simulink model "UAVSim"  (R2025b)
settings: Solver=FixedStepAuto  StartTime=0.0  StopTime=simTime  FixedStep=sampleTime  RelTol=1e-3
values from neighbouring files (symbols this model uses):
  blastParams = [thetaB_rad, phiB_rad, params.c, params.W, params.t0]    [main_optimize.m]
  CM = 0.1    [main_optimize.m]
  CT = m*g/4/rpm_nom^2    [main_optimize.m]
  desRPM = params.motorRPM*ones(4,1)    [main_optimize.m]
  dragConstsBody = -1/2*rho*bodyA*CD    [main_optimize.m]
  dragConstsMotor = -1/2*rho*motorA*CD    [main_optimize.m]
  g = 9.81    [main_optimize.m]
  m = mBody + 4*mMotor + 4*mArm    [main_optimize.m]
  quadDims = [rBody, rMotors, L]    [main_optimize.m]
  RMOTOR_iG = zeros(4,3)    [main_optimize.m]
  rpm2bodyMomentRollPitch = [-L L L -L ... (first row only)    [main_optimize.m]
  sampleTime = 0.0001    [main.m]    (also in main_compare.m)
libraries: aerolibobsolete x1, robotcorelib x1, aerolibutil x1, uavutilslib x1, dspsigops x1
settings Model: PauseTimes=1.23  SnapshotBufferSize=30  SnapshotInterval=1  Creator=root  LastModifiedBy=nkaka
settings DebuggingCC: ReadBeforeWriteMsg=DisableAll  WriteAfterWriteMsg=DisableAll  WriteAfterReadMsg=DisableAll  MultiTaskDSMMsg=none
settings ModelReferenceCC: UpdateModelReferenceTargets=IfOutOfDate
settings SFSimCC: SFSimEcho=off
settings RTWCC: GPUComputeCapability=3.5

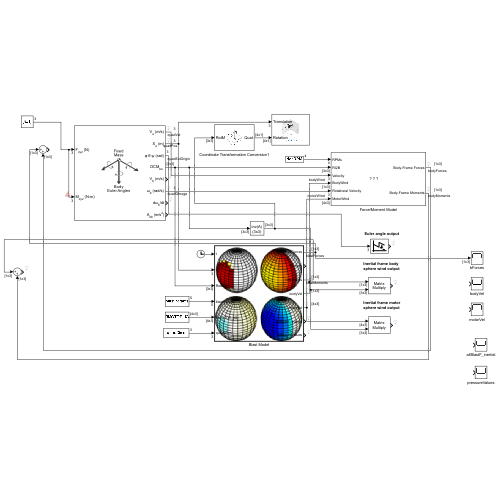
[thumbnail: Simulink's stored preview of the top-level diagram]
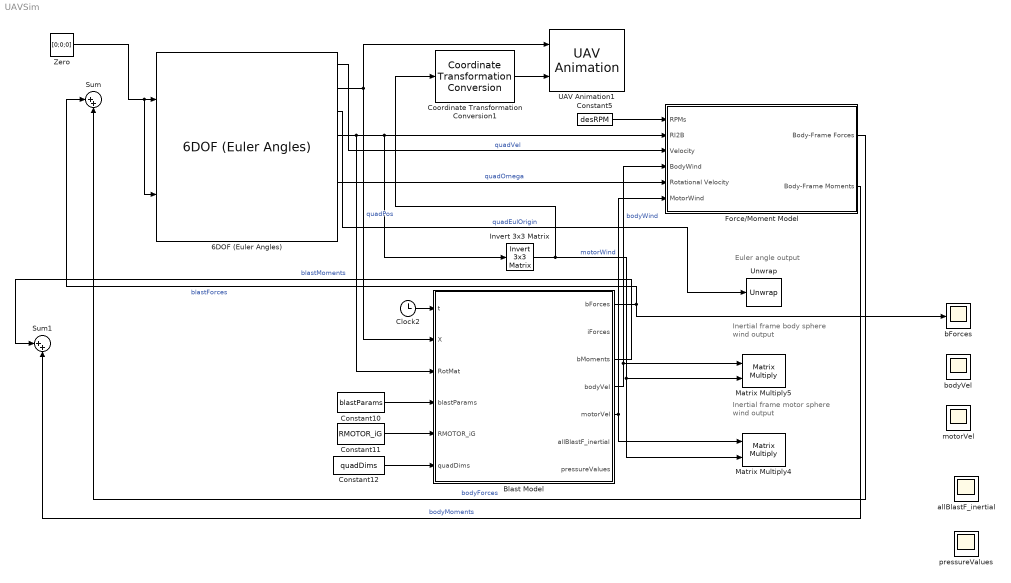
== system UAVSim ==
  note: Euler angle output
  note: Inertial frame body
      | sphere wind output
  note: Inertial frame motor
      | sphere wind output
  6DOF (Euler Angles) : aerolibobsolete/6DOF (Euler Angles)  units=Metric (MKS)  mtype=Fixed  rep=Euler Angles  xme_0=IC  Vm_0=[0 0 0]  eul_0=[0 0 0]  pm_0=[0 0 0]  mass_0=m  mass_e=0.5  mass_f=2.0  inertia=Iquad  inertia_e=eye(3)  inertia_f=2*eye(3)  k_quat=1.0  vre_flag=on  abi_flag=off  aMode=0  xme_statename=''  Vm_statename=''  eul_statename=''  quat_statename=''  pm_statename=''  mass_statename=''
  Blast Model : MATLAB Function  TreatAsAtomicUnit=on
  Clock2 : Clock
  Constant10 : Constant  Value=blastParams
  Constant11 : Constant  Value=RMOTOR_iG
  Constant12 : Constant  Value=quadDims
  Constant5 : Constant  Value=desRPM
  Coordinate Transformation Conversion1 : robotcorelib/Coordinate Transformation Conversion  InputRepresentation=Rotation Matrix  InputEulerSequence=ZYX  ShowTrVecInputPort=on  OutputRepresentation=Quaternion  OutputEulerSequence=ZYX  ShowTrVecOutputPort=on  SimulateUsing=Interpreted execution
      settings: LibrarySourceBlock=uavutilslib/Coordinate Transformation Conversion
  Force/Moment Model : Subsystem
      mask Display: image('simulinkImages/quad3dwithBlast.svg');
  Invert 3x3 Matrix : aerolibutil/Invert  3x3 Matrix
  Matrix Multiply4 : Product  Multiplication=Matrix(*)
  Matrix Multiply5 : Product  Multiplication=Matrix(*)
  Sum : Sum  Inputs=|++
  Sum1 : Sum  Inputs=|++
  UAV Animation1 : uavutilslib/UAV Animation  NumUAV=1  DynamicUAVConfig=off  UAVType=Multirotor  UAVSize=1  UAVColor=[1 0 0]  UAVTrajectoryAlpha=1  InertialZDirection=Down  RotationFormat=Quaternion  DrawMarkers=off  SampleTime=sampleTime
  Unwrap : dspsigops/Unwrap  tol=pi  running=off
  Zero : Constant  Value=[0;0;0]  OutDataTypeStr=Inherit: Inherit via back propagation
  allBlastF_inertial : Scope
      settings: DataLoggingVariableName=ScopeData3
  bForces : Scope
  bodyVel : Scope
  motorVel : Scope
      settings: DataLoggingVariableName=ScopeData2
  pressureValues : Scope
      settings: DataLoggingVariableName=ScopeData4
  wires:
  Blast Model/1(bForces) -> Sum/1, bForces/1  "blastForces"
  6DOF (Euler Angles)/1 -> Force/Moment Model/3(Velocity)  "quadVel"
  Clock2/1 -> Blast Model/1(t)
  6DOF (Euler Angles)/6 -> Force/Moment Model/5(Rotational Velocity)  "quadOmega"
  6DOF (Euler Angles)/2 -> Blast Model/2(X), UAV Animation1/1  "quadPos"
  6DOF (Euler Angles)/3 -> Unwrap/1  "quadEulOrigin"
  6DOF (Euler Angles)/4 -> Force/Moment Model/2(RI2B), Invert 3x3 Matrix/1, Blast Model/3(RotMat)
  Constant10/1 -> Blast Model/4(blastParams)
  Constant11/1 -> Blast Model/5(RMOTOR_iG)
  Constant12/1 -> Blast Model/6(quadDims)
  Constant5/1 -> Force/Moment Model/1(RPMs)
  Invert 3x3 Matrix/1 -> Matrix Multiply4/2, Matrix Multiply5/2, Coordinate Transformation Conversion1/1
  Blast Model/3(bMoments) -> Sum1/1  "blastMoments"
  Force/Moment Model/1(Body-Frame Forces) -> Sum/2  "bodyForces"
  Blast Model/4(bodyVel) -> Force/Moment Model/4(BodyWind), Matrix Multiply5/1  "bodyWind"
  Force/Moment Model/2(Body-Frame Moments) -> Sum1/2  "bodyMoments"
  Blast Model/5(motorVel) -> Matrix Multiply4/1, Force/Moment Model/6(MotorWind)  "motorWind"
  Coordinate Transformation Conversion1/1 -> UAV Animation1/2
  Zero/1 -> 6DOF (Euler Angles)/2, 6DOF (Euler Angles)/1

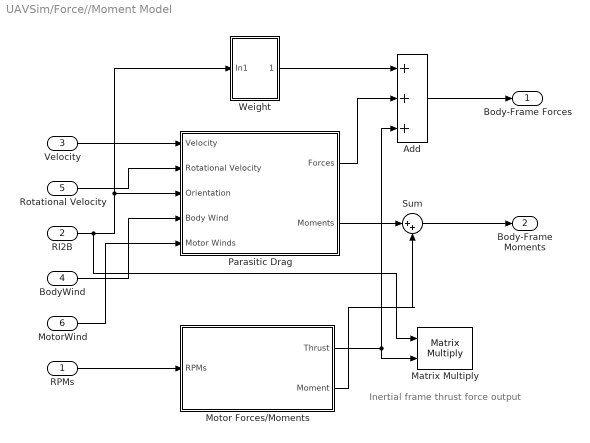
== system UAVSim/Force//Moment Model ==
  note: Inertial frame thrust force output
  RPMs : Inport
  RI2B : Inport  Port=2
  Velocity : Inport  Port=3
  BodyWind : Inport  Port=4
  Rotational Velocity : Inport  Port=5
  MotorWind : Inport  Port=6
  Add : Sum  Inputs=+++
  Matrix Multiply : Product  Multiplication=Matrix(*)
  Motor Forces/Moments : Subsystem
  Parasitic Drag : Subsystem
  Sum : Sum  Inputs=|++
  Weight : Subsystem
  Body-Frame Forces : Outport
  Body-Frame Moments : Outport  Port=2
  wires:
  RPMs/1 -> Motor Forces/Moments/1(RPMs)
  Rotational Velocity/1 -> Parasitic Drag/2(Rotational Velocity)
  Velocity/1 -> Parasitic Drag/1(Velocity)
  MotorWind/1 -> Parasitic Drag/5(Motor Winds)
  BodyWind/1 -> Parasitic Drag/4(Body Wind)
  RI2B/1 -> Weight/1(In1), Parasitic Drag/3(Orientation), Matrix Multiply/1
  Weight/1(Out1) -> Add/1
  Parasitic Drag/1(Forces) -> Add/2
  Parasitic Drag/2(Moments) -> Sum/1
  Motor Forces/Moments/1(Thrust) -> Matrix Multiply/2, Add/3
  Motor Forces/Moments/2(Moment) -> Sum/2
  Add/1 -> Body-Frame Forces/1
  Sum/1 -> Body-Frame Moments/1

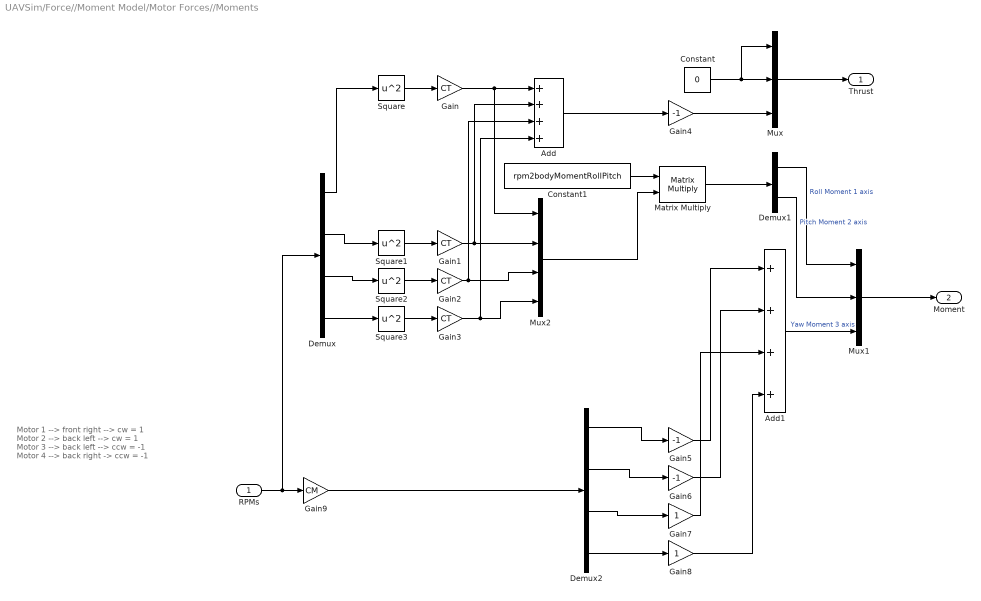
== system UAVSim/Force//Moment Model/Motor Forces//Moments ==
  note: Motor 1 --> front right --> cw = 1
      | Motor 2 --> back left --> cw = 1
      | Motor 3 --> back left --> ccw = -1
      | Motor 4 --> back right -> ccw = -1
  RPMs : Inport
  Add : Sum  Inputs=++++
  Add1 : Sum  Inputs=++++
  Constant : Constant  Value=0
  Constant1 : Constant  Value=rpm2bodyMomentRollPitch
  Demux : Demux
  Demux1 : Demux  Outputs=2
  Demux2 : Demux
  Gain{,1..3} (4 alike) : Gain  Gain=CT
  Gain4 : Gain  Gain=-1
  Gain5 : Gain  Gain=-1
  Gain6 : Gain  Gain=-1
  Gain7 : Gain
  Gain8 : Gain
  Gain9 : Gain  Gain=CM
  Matrix Multiply : Product  Multiplication=Matrix(*)
  Mux : Mux  Inputs=3
  Mux1 : Mux  Inputs=3
  Mux2 : Mux
  Square{,1..3} (4 alike) : Math  Operator=square
  Thrust : Outport
  Moment : Outport  Port=2
  wires:
  RPMs/1 -> Demux/1, Gain9/1
  Demux/1 -> Square/1
  Demux/2 -> Square1/1
  Demux2/1 -> Gain5/1
  Demux/3 -> Square2/1
  Square2/1 -> Gain2/1
  Gain9/1 -> Demux2/1
  Constant/1 -> Mux/2, Mux/1
  Demux/4 -> Square3/1
  Square/1 -> Gain/1
  Square1/1 -> Gain1/1
  Gain/1 -> Mux2/1, Add/1
  Square3/1 -> Gain3/1
  Gain1/1 -> Mux2/2, Add/2
  Gain2/1 -> Add/3, Mux2/3
  Gain3/1 -> Add/4, Mux2/4
  Add/1 -> Gain4/1
  Constant1/1 -> Matrix Multiply/1
  Mux2/1 -> Matrix Multiply/2
  Demux2/2 -> Gain6/1
  Demux2/3 -> Gain7/1
  Demux2/4 -> Gain8/1
  Gain4/1 -> Mux/3
  Matrix Multiply/1 -> Demux1/1
  Demux1/2 -> Mux1/2  "Pitch Moment 2 axis"
  Gain5/1 -> Add1/1
  Gain6/1 -> Add1/2
  Gain7/1 -> Add1/3
  Gain8/1 -> Add1/4
  Mux/1 -> Thrust/1
  Demux1/1 -> Mux1/1  "Roll Moment 1 axis"
  Add1/1 -> Mux1/3  "Yaw Moment 3 axis"
  Mux1/1 -> Moment/1

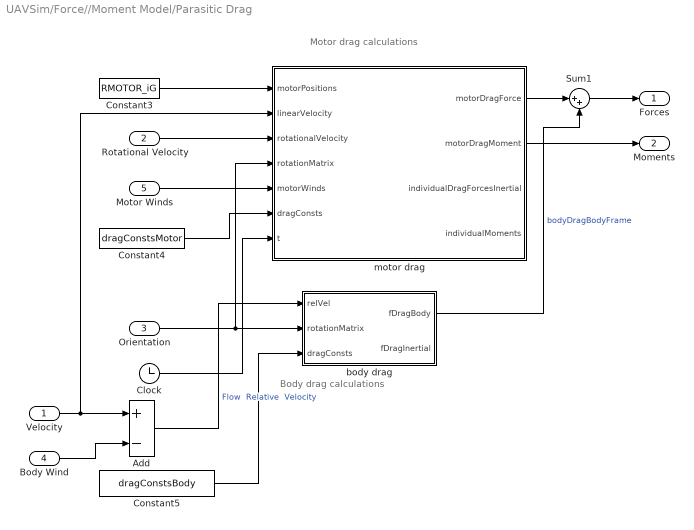
== system UAVSim/Force//Moment Model/Parasitic Drag ==
  note: Motor drag calculations
  note: Body drag calculations
  Velocity : Inport
  Rotational Velocity : Inport  Port=2
  Orientation : Inport  Port=3
  Body Wind : Inport  Port=4
  Motor Winds : Inport  Port=5
  Add : Sum  Inputs=+-
  Clock : Clock
  Constant3 : Constant  Value=RMOTOR_iG
  Constant4 : Constant  Value=dragConstsMotor
  Constant5 : Constant  Value=dragConstsBody
  Sum1 : Sum  Inputs=|++
  body drag : MATLAB Function  TreatAsAtomicUnit=on
  motor drag : MATLAB Function  TreatAsAtomicUnit=on
  Forces : Outport
  Moments : Outport  Port=2
  wires:
  Orientation/1 -> motor drag/4(rotationMatrix), body drag/2(rotationMatrix)
  Velocity/1 -> Add/1, motor drag/2(linearVelocity)
  Constant4/1 -> motor drag/6(dragConsts)
  Motor Winds/1 -> motor drag/5(motorWinds)
  body drag/1(fDragBody) -> Sum1/2  "bodyDragBodyFrame"
  Body Wind/1 -> Add/2
  Clock/1 -> motor drag/7(t)
  Constant5/1 -> body drag/3(dragConsts)
  Rotational Velocity/1 -> motor drag/3(rotationalVelocity)
  Constant3/1 -> motor drag/1(motorPositions)
  Add/1 -> body drag/1(relVel)  "Flow  Relative  Velocity"
  motor drag/1(motorDragForce) -> Sum1/1
  motor drag/2(motorDragMoment) -> Moments/1
  Sum1/1 -> Forces/1

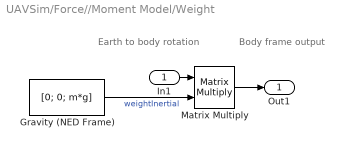
== system UAVSim/Force//Moment Model/Weight ==
  note: Earth to body rotation
  note: Body frame output
  In1 : Inport
  Gravity (NED Frame) : Constant  Value=[0; 0; m*g]
  Matrix Multiply : Product  Multiplication=Matrix(*)
  Out1 : Outport
  wires:
  Gravity (NED Frame)/1 -> Matrix Multiply/2  "weightInertial"
  In1/1 -> Matrix Multiply/1
  Matrix Multiply/1 -> Out1/1

== matlab function UAVSim/Blast Model ==
  data: t input; X input double; bForces output double [-500000..500000]; iForces output; RotMat input; blastParams input; RMOTOR_iG input; quadDims input; bMoments output double [-500000..500000]; bodyVel output double; motorVel output double; allBlastF_inertial output; pressureValues output
function [bForces, iForces, bMoments, bodyVel, motorVel, allBlastF_inertial, pressureValues] = blastFMCalc(t, X, RotMat, blastParams, RMOTOR_iG, quadDims)
%% Inputs:
% t = current sim time
% X = current quad position
% RotMat = current quad orientation matrix earth to body frame
% blastParams = [Time of hit, Overpressure, theta, psi, tau, c] = [t, Ps, theta, psi, tau, c]
% RMOTOR_iG = Motor positions = [rBody, rMotors, rMotors, rMotors, rMotors]
% quadDims = Quadrotor dimensions = [rBody, rMotors, L]
% onOff = toggle for enabling the blasts in the simulink simulation

%% Initialize outputs
bForces = zeros(1,3);
iForces = zeros(1,3);
bMoments = zeros(1,3);
bodyVel = zeros(1,3);
motorVel = zeros(4,3);
allBlastF_inertial = zeros(5,3);
pressureValues = zeros(5,100);
onOffPressure = 1;
onOffVelocity = 1;
mach2ms = 343;

%% Unpack quadrotor dimensions
rBody = quadDims(1);
rMotors = quadDims(2);

%% Make the rotation matrix more clear
Rb2i = RotMat';
Ri2b = RotMat;

%% Get blast parameters
t0 = blastParams(5);
theta = blastParams(1); % Elevation
phi = blastParams(2); % Azimuth
ccccccccc = blastParams(3);
W = blastParams(4);

% Best fit c function
% cF = 
% 
%      General model Power2:
%      cF(x) = a*x^b+c
%      Coefficients (with 95% confidence bounds):
%        a =        1698  (1687, 1709)
%        b =     -0.6454  (-0.6496, -0.6413)
%        c =       73.96  (67.94, 79.98)
function c = cF(x)
    c = 1698*abs(x)^(-0.6454) + 73.96;
end

% Calculate vector for orientation of the blast, opposite of NED to get the intended effect
vec = [sin(phi)*cos(theta), sin(phi)*sin(theta), cos(phi)]*Ri2b;

%% Setup Sadovskiy models for tau and Ps
function [sadPs, sadTau] = sadovskiy(WW,RR)
% Check that RR is positive
assert(RR >= 0);

% Set common consts
crW = WW^(1/3);
kgcmsq2pa = 98066.5;

% Calculate values from Sadovisky
sadTau = nthroot(WW,6)*sqrt(RR)/1000; % converted to seconds
sadPs = (0.95*(crW/RR) + 3.9*((crW/RR)^2) + 13*((crW/RR)^3))*kgcmsq2pa;
end

%% Setup heaviside function since the default matlab one won't work with code gen
function H = heavisideFcn(X)
    % https://en.wikipedia.org/wiki/Heaviside_step_function
    H = zeros(size(X));
    for iii = 1:length(X)
        if X(iii) >= 0
            H(iii) = 1;
        % else
        %     H(i) = 0;
        end
    end
end

%% Setup a rounding function for rounding to a particular decimal place with code-gen
function out = round2Digits(in,decs)
% https://www.mathworks.com/matlabcentral/answers/17598-how-to-convert-a-string-to-int
roundingNum = str2double(append('1',repmat(['0'],1,decs-1)));
out = round(in.*roundingNum)./roundingNum;
end

%% Setup the dewey parameter interpolation functions
function [v,alpha,beta,a,tstar] = deweyParams(scaledDist)
%% Function info:
% Inputs:
%      scaledDist = d/S = double
%          d = distance from blast
%          S = (W*P0/P)^(1/3)
%               W = weight of explosive used in blast
%               P0 = standard pressure = 101.325
%               P = ambient pressure
%
% Outputs:
%      v = peak velocity (m/s), converted from mach
%      alpha = unitless fitted parameter
%      beta = unitless fitted parameter
%      a = unitless fitted parameter
%      tstar = unitless fitted parameter

%% Setup the dewey parameter interpolation functions
% Set functions for interpolating the parameters, with their derivatives
function out = vMachFcn(xx,option)
    if option == 1
        vMach1 = 6.38*xx^-1.51;
        out = vMach1;
    elseif option == 2
        vMachDer = (-1.51*6.38)*xx^(-1.51-1);
        out = vMachDer;
    else
        error('Choose a valid output option')
    end
end

function out = alphaFcn(xx, option)
    if option == 1
        alpha1 = 1.5*xx^-0.926; % power series
        out = alpha1;
    elseif option == 2
        alphaDer = (-0.926*1.5)*xx^(-0.926-1);
        out = alphaDer;
    else
        error('Choose a valid output option')
    end
end

function out = betaFcn(xx,option)
    if option == 1
        beta1 = 1.64*xx^(-0.241); % Power
        out = beta1;
    elseif option == 2
        betaDer = (-0.241*1.64)*xx^(-0.241-1);
        out = betaDer;
    else
        error('Choose a valid output option')
    end
end

function out = aFcn(xx,option)
    if option == 1
        a1 = 1.95*xx^-1.02; % power series
        out = a1;
    elseif option == 2
        aDer = (-1.02*1.95)*xx^(-1.02-1);
        out = aDer;
    else
        error('Choose a valid output option')
    end
end

function out = tstarFcn(xx,option)
    if option == 1
        tstar1 = -0.326+0.93*log(max(1e-10, xx)); % Log
        out = tstar1;
    elseif option == 2
        tstarDer = 0.93/xx;
        out = tstarDer;
    else
        error('Choose a valid output option')
    end
end

% Set point to swtich from fitted curves to linear extrapolation for power series fits
xpt = 1.983489191;

% Set scaleDist to x for readability
xx = scaledDist;

% Peak velocity value - power series/ linear piecewise interpolation
if xx >= xpt
    % Regular interp function
    vMach = vMachFcn(xx,1);
else
    % Linear interp function
    yVal = vMachFcn(xpt,1);
    slope = vMachFcn(xpt,2);
    yIntercept = yVal - slope*xpt;
    vMach = slope*xx + yIntercept;
end
v = vMach;

% Alpha - power series/ linear piecewise interpolation
if xx >= xpt
    % Regular interp function
    alpha = alphaFcn(xx,1);
else
    % Linear interp function
    yVal = alphaFcn(xpt,1);
    slope = alphaFcn(xpt,2);
    yIntercept = yVal - slope*xpt;
    alpha = slope*xx + yIntercept;
end

% Beta - linear interpolation
if xx >= xpt
    % Regular interp function
    beta = betaFcn(xx,1);
else
    % Linear interp function
    yVal = betaFcn(xpt,1);
    slope = betaFcn(xpt,2);
    yIntercept = yVal - slope*xpt;
    beta = slope*xx + yIntercept;
end

% a - power series/ linear piecewise interpolation
if xx >= xpt
    % Regular interp function
    a = aFcn(xx,1);
else
    % Linear interp function
    yVal = aFcn(xpt,1);
    slope = aFcn(xpt,2);
    yIntercept = yVal - slope*xpt;
    a = slope*xx + yIntercept;
end

% tstar - linear interpolation
if xx >= xpt
    % Regular interp function
    tstar = tstarFcn(xx,1);
else
    % Linear interp function
    yVal = tstarFcn(xpt,1);
    slope = tstarFcn(xpt,2);
    yIntercept = yVal - slope*xpt;
    tstar = slope*xx + yIntercept;
end

end

%% Update outputs if onOff is true
if onOffPressure == 1
    %% Set sphere sizes and distances from center of blast
    d = -vecnorm(X);
    x = [linspace(-rBody,rBody);
         linspace(-rMotors,rMotors);
         linspace(-rMotors,rMotors);
         linspace(-rMotors,rMotors);
         linspace(-rMotors,rMotors)] + d;
    n = height(x);
    ds = zeros(n,1);
    for i = 1:n
        if i == 1
            ds(i) = vecnorm(X');
        else
            ds(i) = vecnorm(X'-RMOTOR_iG(i-1,:));
        end
    end

    %% Get the forces based on the desired times and overpressure values
    Fp = zeros(n,3);
    V = zeros(n,3);

    %% Get curret pressure at x1
    pp = zeros(size(x));
    for j = 1:n
        % Set radius
        if j == 1
            R = rBody;
            x0 = d - R;
        else
            R = rMotors;
            dTmp = vecnorm(X'-RMOTOR_iG(j-1,:));
            x0 = -dTmp - R;
        end
        [Ps, tau] = sadovskiy(W,ds(j));
    
        % Calculate pressure for this time step
        % val = t-(x(j,:)-x0)/ccccccccc;
        val = t-(x(j,:)-x0)/cF(d);
        Dt = val-t0;
        expr = Dt./tau;
        hval = heavisideFcn(Dt);
        pp(j,:) = Ps.*exp(-expr).*(1-expr).*hval;

        %% Calculate velocity based on modified Dewey model
        if onOffVelocity == 1
            % Get Dt
            ti = t;
            DT = ti-t0;
        
            % Calcualte scaled distance
            % val = t-(x(j,:)-x0)/ccccccccc;
            val = t-(x(j,:)-x0)/cF(d);
            Dt = val-t0; 
            hval = heavisideFcn(Dt);
            S = W^(1/3);
            scaledDist = ds(j)/S;
            % hval = heavisideFcn(ti-t0);
            % scaledTime = ccccccccc*DT/S;
            scaledTime = cF(d)*DT/S;

            % Get dewey params
            [Vs_i, alpha_i, beta_i, a_i, ~] = deweyParams(scaledDist);

            % Calculate velocity
            logVal = 1 + beta_i*scaledTime;
            if logVal < 0
                1;
            end
            % V(j,:) = (mach2ms * ((Vs_i*(1-beta_i*scaledTime) * exp(-alpha_i*scaledTime) + a_i*log(1 + beta_i*scaledTime)) * exp(-scaledTime)*ceil(sum(hval)/length(hval))))*vec;
            logVal = max(1e-10, 1 + beta_i*scaledTime);
            V(j,:) = (mach2ms * ((Vs_i*(1-beta_i*scaledTime) * exp(-alpha_i*scaledTime) + a_i*log(logVal)) * exp(-scaledTime)*ceil(sum(hval)/length(hval))))*vec;
           
        end
        if any(isnan(V))
            1;
        end
        roundedV = real(round2Digits(V,5)); % added real(.) here because otherwise simulink thinks that V could be complex due to it inheriting a variable that was once square rooted.............
        if any(isnan(roundedV))
            1;
        end
    end
    pressureValues = pp;
    
    %% Get current force due to pressure based on x1
    eps = 0.0000001;
    for j = 1:n
        % Set radius
        if j == 1
            R = rBody;
        else
            R = rMotors;
        end
    
        % Set current x and pp values
        currX = x(j,:);
        currPP = pp(j,:);

        % Calculate force
        sqrtVal = (R + eps)^2+(currX-d).^2;
        if any(sqrtVal < 0)
            1;
        end
        Fp(j,:) = ((trapz(currX-d,currPP.*(currX-d).*sqrt(sqrtVal))*-pi/R).*vec);
    end

    %% Output the velocities
    bodyVel = roundedV(1,:);
    motorVel = roundedV(2:5,:);

    %% Calculate total force due to the blast
    bForces = sum(Fp,1);
    iForces = bForces*Rb2i;
    
    %% Calculate resultant moment from blast
    Mblast = zeros(n-1,3);
    for j = 2:n
        Mblast(j-1,:) = cross(RMOTOR_iG(j-1,:),Fp(j,:));
    end
    bMoments = sum(Mblast,1);

    % Output full matrix of blast forces and moments
    allBlastF_inertial = Fp*Rb2i;
end

assert(~anynan(bForces) || allfinite(bForces))
assert(~anynan(iForces) || allfinite(iForces))
assert(~anynan(bMoments) || allfinite(bMoments))
assert(~anynan(bodyVel) || allfinite(bodyVel))
assert(~anynan(motorVel) || allfinite(motorVel))
assert(~anynan(allBlastF_inertial) || allfinite(allBlastF_inertial))


end

== matlab function UAVSim/Force//Moment Model/Parasitic Drag/motor drag ==
  data: motorPositions input; motorDragForce output; linearVelocity input; rotationalVelocity input; rotationMatrix input; motorDragMoment output; motorWinds input; dragConsts input; t input; individualDragForcesInertial output; individualMoments output
function [motorDragForce,motorDragMoment,individualDragForcesInertial,individualMoments] = motorDragCalc(motorPositions, linearVelocity, rotationalVelocity, rotationMatrix, motorWinds, dragConsts, t)
% Function to calculate the drag force and moments for the motors
% Inputs: 
%      motorPositions = Matrix of four position vectors denoting the position of each motor relative to the body (4,3)
%      linearVelocity = Linear velocity vector of the drone (1,3)
%      rotationalVelocity = Rotational velocity vector of the drone (1,3)
%      rotationMatrix = Orientation matrix of the drone (3,3) - inertial to body frame
%      motorWinds = wind experienced at each motor position (4,3)
%      dragConsts = -1/2 * rho * C_D * motorA
%
% Outputs:
%      motorDragForce = vector of total drag force on all motors (BODY FRAME)
%      motorDragMoment = vector of total drag moment caused by the wind-relative velocity on each motor (BODY FRAME)

%% Set output sizes
motorDragForce = zeros(1,3);
motorDragMoment = zeros(1,3);
individualDragForcesInertial = zeros(4,3);
individualMoments = zeros(4,3);

%% Set variables for readability
v = linearVelocity;
W = rotationalVelocity;
Rb2i = rotationMatrix';
Ri2b = rotationMatrix;
r_iG = motorPositions;

%% Calculate individual motor velocities
% Inertial velocity at each element
vmotor_iG = zeros(4,3);
vRelmotor_iG = zeros(4,3);
fDrag = zeros(4,3);
mDrag = zeros(4,3);
for i = 1:4
    vmotor_iG(i,:) = (v + (Rb2i*cross(r_iG(i,:),W)'));
    vRelmotor_iG(i,:) = vmotor_iG(i,:) - (Ri2b*motorWinds(i,:)')';
    vTmp = vRelmotor_iG(i,:);
    vecNorm = vecnorm(vTmp);

    % Calculate drag in the inertial frame, but output in the body frame
    fDrag(i,:) = (Ri2b*(dragConsts*vecNorm.*vTmp'))';

    % Calculate the drag momenet in the body frame
    mDrag(i,:) = cross(fDrag(i,:),r_iG(i,:));
end

%% Output force and moments
motorDragForce = sum(fDrag,1);
individualDragForcesInertial = fDrag*Rb2i;
motorDragMoment = sum(mDrag,1);
individualMoments = mDrag;

end

== matlab function UAVSim/Force//Moment Model/Parasitic Drag/body drag ==
  data: relVel input; fDragBody output; rotationMatrix input; dragConsts input; fDragInertial output
function [fDragBody, fDragInertial] = bodyDragCalc(relVel, rotationMatrix, dragConsts)
% Initialize
fDragBody = zeros(1,3);
fDragInertial = zeros(1,3);

% Unpack
Rb2i = rotationMatrix';
Ri2b = rotationMatrix;

% Calculate
vecNorm = sqrt(sum(conj(relVel).*relVel));
fDragBody = dragConsts*vecNorm.*relVel*Rb2i;
fDragInertial = fDragBody*Ri2b;

end
